simulink model "gm_whdlOFDMTx"  (R2022b)
settings: Solver=FixedStepDiscrete  StartTime=0.0  StopTime=0  RelTol=1e-3
model workspace (MATLAB code in the model file):
  | config = whdlexamples.OFDMTxParameters();
  | fftLen = config.fftLen;
  | subC = config.subC;
  | cpLen = config.cpLen;
  | fs = config.fs;
  | NSS = config.NSS;
  | NRS = config.NRS;
  | NHeader = config.NHeader;
  | NData = config.NData;
  | NSymPerF = config.NSymPerF;
  | ssSymbol = config.ssSymbol;
  | rsSymbol = config.rsSymbol;
  | NHeaderBits = config.NHeaderBits;
  | headerCRCBool = config.headerCRCBool;
  | headerConvK = config.headerConvK;
  | headerConvCode = config.headerConvCode;
  | pilotValPerSym = config.pilotValPerSym;
  | pilotLen = config.pilotLen;
  | dataCRCPoly = config.dataCRCPoly;
  | dataCRCBool = config.dataCRCBool;
  | dataCRCLen = config.dataCRCLen;
  | dataConvK = config.dataConvK;
  | dataConvCode = config.dataConvCode;
  | scramInit = config.scramInit;
  | firCoeff = config.firCoeff;
  | rateFac1 = config.rateFac1;
  | rateFac2 = config.rateFac2;
  | headerLat = config.headerLat;
  | headerTime = config.headerTime;
  | preambleInd = config.preambleInd;
  | headerDataInd = config.headerDataInd;
  | trBlkSize = config.trBlkSize;
  | randOFDM = config.randOFDM;
  | headerIntrlvMaxBlkSize = config.headerIntrlvMaxBlkSize;
  | headerIntrlvNColumns   = config.headerIntrlvNColumns;
  | dataIntrlvMaxBlkSize   = config.dataIntrlvMaxBlkSize;
  | dataIntrlvNColumns     = config.dataIntrlvNColumns;
  | clear config
libraries: hdlsllib x49, simulink x22, dspsigops x11, whdlmod x3, whdledac x3, whdlutilities x2, commhdlcrc x2, dsphdlfiltering2 x1
(part 3 of 4)

== system gm_whdlOFDMTx/Frame Generator/Header/Interleaver/Read Logic/Generate Base Read Address ==
  readStart : Inport  OutDataTypeStr=boolean  PortDimensions=1  SampleTime=2.44140625e-07
  Constant1 : Constant  Value=0  OutDataTypeStr=fixdt(0,nextpow2(maxBlkSize+1),0)  SampleTime=-1
  Constant5 : Constant  Value=maxBlkSize  OutDataTypeStr=fixdt(0,nextpow2(maxBlkSize+1),0)  SampleTime=-1
  Logical Operator7 : Logic  Operator=NOT  IconShape=distinctive  AllPortsSameDT=off  OutDataTypeStr=boolean
  Switch1 : Switch  Criteria=u2 ~= 0  SaturateOnIntegerOverflow=off  InputSameDT=off
  Unit Delay Enabled Synchronous2 : hdlsllib/Discrete/Unit Delay Enabled Synchronous  InitialCondition=1  SampleTime=-1
  baseAddr : Outport  SampleTime=2.44140625e-07
  wires:
  readStart/1 -> Unit Delay Enabled Synchronous2/2
  Constant1/1 -> Switch1/3
  Constant5/1 -> Switch1/1
  Logical Operator7/1 -> Unit Delay Enabled Synchronous2/1
  Switch1/1 -> baseAddr/1
  Unit Delay Enabled Synchronous2/1 -> Switch1/2, Logical Operator7/1

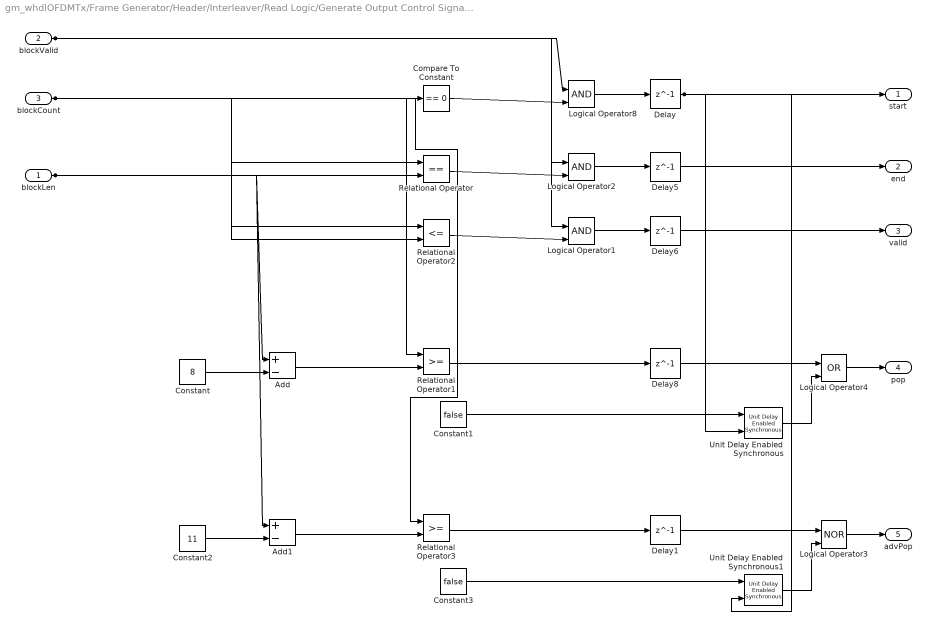
== system gm_whdlOFDMTx/Frame Generator/Header/Interleaver/Read Logic/Generate Output Control Signals ==
  blockLen : Inport  OutDataTypeStr=fixdt(0, 7, 0)  PortDimensions=1  SampleTime=2.44140625e-07
  blockValid : Inport  Port=2  OutDataTypeStr=boolean  PortDimensions=1  SampleTime=2.44140625e-07
  blockCount : Inport  Port=3  OutDataTypeStr=fixdt(0, 7, 0)  PortDimensions=1  SampleTime=2.44140625e-07
  Add : Sum  Inputs=+-
  Add1 : Sum  Inputs=+-
  Compare To Constant : simulink/Logic and Bit Operations/Compare To Constant  relop===  const=0  OutDataTypeStr=boolean
  Constant : Constant  Value=8  OutDataTypeStr=fixdt(0,nextpow2(8+1),0)  SampleTime=-1
  Constant1 : Constant  Value=false  SampleTime=-1
  Constant2 : Constant  Value=11  OutDataTypeStr=fixdt(0,nextpow2(11+1),0)  SampleTime=-1
  Constant3 : Constant  Value=false  SampleTime=-1
  Delay{,1,5..6,8} (5 alike) : Delay  DelayLength=1
  Logical Operator1 : Logic  IconShape=distinctive  AllPortsSameDT=off  OutDataTypeStr=boolean
  Logical Operator2 : Logic  IconShape=distinctive  AllPortsSameDT=off  OutDataTypeStr=boolean
  Logical Operator3 : Logic  Operator=NOR  IconShape=distinctive  AllPortsSameDT=off  OutDataTypeStr=boolean
  Logical Operator4 : Logic  Operator=OR  IconShape=distinctive  AllPortsSameDT=off  OutDataTypeStr=boolean
  Logical Operator8 : Logic  IconShape=distinctive  AllPortsSameDT=off  OutDataTypeStr=boolean
  Relational Operator : RelationalOperator  Operator===  OutDataTypeStr=boolean  InputSameDT=off
  Relational Operator1 : RelationalOperator  OutDataTypeStr=boolean  InputSameDT=off
  Relational Operator2 : RelationalOperator  Operator=<=  OutDataTypeStr=boolean  InputSameDT=off
  Relational Operator3 : RelationalOperator  OutDataTypeStr=boolean  InputSameDT=off
  Unit Delay Enabled Synchronous : hdlsllib/Discrete/Unit Delay Enabled Synchronous  InitialCondition=1  SampleTime=-1
  Unit Delay Enabled Synchronous1 : hdlsllib/Discrete/Unit Delay Enabled Synchronous  InitialCondition=1  SampleTime=-1
  start : Outport  SampleTime=2.44140625e-07
  end : Outport  Port=2  SampleTime=2.44140625e-07
  valid : Outport  Port=3  SampleTime=2.44140625e-07
  pop : Outport  Port=4  SampleTime=2.44140625e-07
  advPop : Outport  Port=5  SampleTime=2.44140625e-07
  wires:
  blockLen/1 -> Relational Operator2/2, Relational Operator/2, Add1/1, Add/1
  blockValid/1 -> Logical Operator8/1, Logical Operator2/1, Logical Operator1/1
  blockCount/1 -> Relational Operator3/1, Relational Operator2/1, Relational Operator1/1, Relational Operator/1, Compare To Constant/1
  Add/1 -> Relational Operator1/2
  Add1/1 -> Relational Operator3/2
  Compare To Constant/1 -> Logical Operator8/2
  Constant/1 -> Add/2
  Constant1/1 -> Unit Delay Enabled Synchronous/1
  Constant2/1 -> Add1/2
  Constant3/1 -> Unit Delay Enabled Synchronous1/1
  Delay/1 -> Unit Delay Enabled Synchronous1/2, Unit Delay Enabled Synchronous/2, start/1
  Delay1/1 -> Logical Operator3/1
  Delay5/1 -> end/1
  Delay6/1 -> valid/1
  Delay8/1 -> Logical Operator4/1
  Logical Operator1/1 -> Delay6/1
  Logical Operator2/1 -> Delay5/1
  Logical Operator3/1 -> advPop/1
  Logical Operator4/1 -> pop/1
  Logical Operator8/1 -> Delay/1
  Relational Operator/1 -> Logical Operator2/2
  Relational Operator1/1 -> Delay8/1
  Relational Operator2/1 -> Logical Operator1/2
  Relational Operator3/1 -> Delay1/1
  Unit Delay Enabled Synchronous/1 -> Logical Operator4/2
  Unit Delay Enabled Synchronous1/1 -> Logical Operator3/2

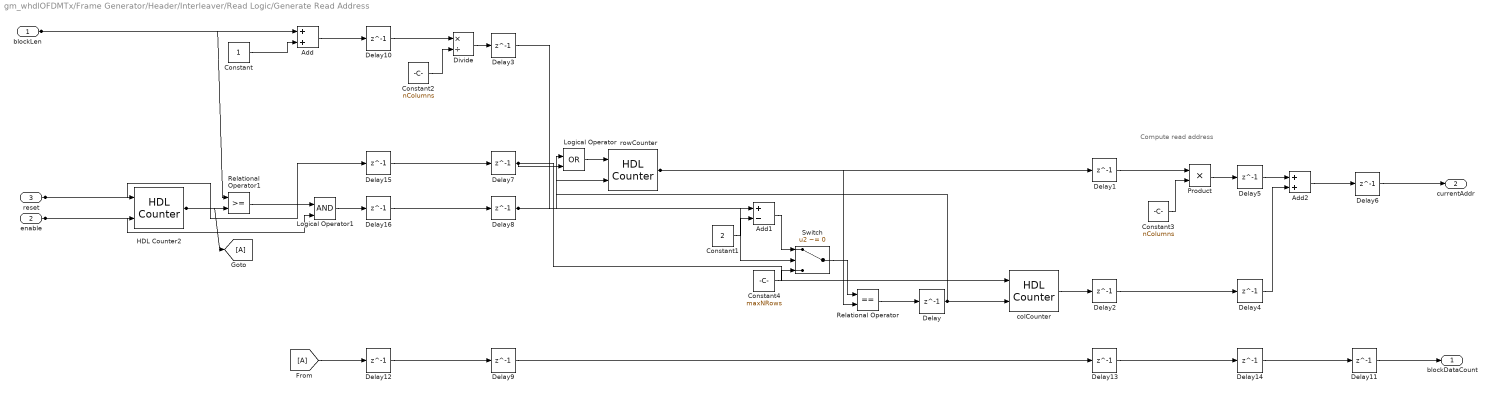
== system gm_whdlOFDMTx/Frame Generator/Header/Interleaver/Read Logic/Generate Read Address ==
  note: Compute read address
  blockLen : Inport  OutDataTypeStr=fixdt(0, 7, 0)  PortDimensions=1  SampleTime=2.44140625e-07
  enable : Inport  Port=2  OutDataTypeStr=boolean  PortDimensions=1  SampleTime=2.44140625e-07
  reset : Inport  Port=3  OutDataTypeStr=boolean  PortDimensions=1  SampleTime=2.44140625e-07
  Add : Sum
  Add1 : Sum  Inputs=+-  OutDataTypeStr=Inherit: Inherit via back propagation
  Add2 : Sum  OutDataTypeStr=fixdt(0,nextpow2(maxBlkSize),0)
  Constant : Constant  OutDataTypeStr=fixdt(0,1,0)  SampleTime=-1
  Constant1 : Constant  Value=2  OutDataTypeStr=fixdt(0,2,0)  SampleTime=-1
  Constant2 : Constant  Value=nColumns  OutDataTypeStr=fixdt(0,nextpow2(nColumns+1),0)  SampleTime=-1
  Constant3 : Constant  Value=nColumns  OutDataTypeStr=fixdt(0,nextpow2(nColumns+1),0)  SampleTime=-1
  Constant4 : Constant  Value=maxNRows  OutDataTypeStr=Inherit: Inherit via back propagation  SampleTime=-1
  Delay{,1..16} (17 alike) : Delay  DelayLength=1
  Divide : Product  Inputs=*/  OutDataTypeStr=fixdt(0,nextpow2(maxNRows+1),0)  RndMeth=Zero  SaturateOnIntegerOverflow=on
  From : From
  Goto : Goto
  HDL Counter2 : hdlsllib/Sources/HDL Counter  CountType=Count limited  CountInit=0  CountStep=1  CountMax=maxBlkSize  CountFromType=Initial value  CountFrom=0  CountResetPort=on  CountLoadPort=off  CountEnbPort=on  CountDirPort=off  CountHitOutputPort=off  CountDataType=Unsigned  CountWordLen=nextpow2(maxBlkSize+1)  CountFracLen=0  CountSampTime=1
  Logical Operator : Logic  Operator=OR  IconShape=distinctive  AllPortsSameDT=off  OutDataTypeStr=boolean
  Logical Operator1 : Logic  IconShape=distinctive  AllPortsSameDT=off  OutDataTypeStr=boolean
  Product : Product  OutDataTypeStr=fixdt(0,nextpow2(maxBlkSize),0)
  Relational Operator : RelationalOperator  Operator===  OutDataTypeStr=boolean  InputSameDT=off
  Relational Operator1 : RelationalOperator  OutDataTypeStr=boolean  InputSameDT=off
  Switch : Switch  Criteria=u2 ~= 0  SaturateOnIntegerOverflow=off  InputSameDT=off
  colCounter : hdlsllib/Sources/HDL Counter  CountType=Count limited  CountInit=0  CountStep=1  CountMax=nColumns -1  CountFromType=Initial value  CountFrom=0  CountResetPort=on  CountLoadPort=off  CountEnbPort=on  CountDirPort=off  CountHitOutputPort=off  CountDataType=Unsigned  CountWordLen=nextpow2(nColumns)  CountFracLen=0  CountSampTime=1
  rowCounter : hdlsllib/Sources/HDL Counter  CountType=Count limited  CountInit=0  CountStep=1  CountMax=maxNRows -1  CountFromType=Initial value  CountFrom=0  CountResetPort=on  CountLoadPort=off  CountEnbPort=on  CountDirPort=off  CountHitOutputPort=off  CountDataType=Unsigned  CountWordLen=nextpow2(maxNRows+1)  CountFracLen=0  CountSampTime=1
  blockDataCount : Outport  SampleTime=2.44140625e-07
  currentAddr : Outport  Port=2  SampleTime=2.44140625e-07
  wires:
  blockLen/1 -> Relational Operator1/1, Add/1
  enable/1 -> Logical Operator1/2, HDL Counter2/2
  reset/1 -> Delay15/1, HDL Counter2/1
  Add/1 -> Delay10/1
  Add1/1 -> Switch/1
  Add2/1 -> Delay6/1
  Constant/1 -> Add/2
  Constant1/1 -> Add1/2
  Constant2/1 -> Divide/2
  Constant3/1 -> Product/2
  Constant4/1 -> Switch/3
  Delay/1 -> Logical Operator/1, colCounter/2
  Delay1/1 -> Product/1
  Delay10/1 -> Divide/1
  Delay11/1 -> blockDataCount/1
  Delay12/1 -> Delay9/1
  Delay13/1 -> Delay14/1
  Delay14/1 -> Delay11/1
  Delay15/1 -> Delay7/1
  Delay16/1 -> Delay8/1
  Delay2/1 -> Delay4/1
  Delay3/1 -> Add1/1
  Delay4/1 -> Add2/2
  Delay5/1 -> Add2/1
  Delay6/1 -> currentAddr/1
  Delay7/1 -> Logical Operator/2, colCounter/1
  Delay8/1 -> Switch/2, rowCounter/2
  Delay9/1 -> Delay13/1
  Divide/1 -> Delay3/1
  From/1 -> Delay12/1
  HDL Counter2/1 -> Relational Operator1/2, Goto/1
  Logical Operator/1 -> rowCounter/1
  Logical Operator1/1 -> Delay16/1
  Product/1 -> Delay5/1
  Relational Operator/1 -> Delay/1
  Relational Operator1/1 -> Logical Operator1/1
  Switch/1 -> Relational Operator/1
  colCounter/1 -> Delay2/1
  rowCounter/1 -> Relational Operator/2, Delay1/1

== system gm_whdlOFDMTx/Frame Generator/Header/Interleaver/Read Logic/MATLAB Function ==
  trigger : Inport  OutDataTypeStr=boolean  PortDimensions=1  SampleTime=2.44140625e-07
  MATLAB Function : MATLAB Function  TreatAsAtomicUnit=on  mask{nClocks=maxBlkSize}
      mask prompts: nClocks "Number of clocks to hold:"
  out : Outport  SampleTime=2.44140625e-07  VectorParamsAs1DForOutWhenUnconnected=off
  wires:
  trigger/1 -> MATLAB Function/1(trigger)
  MATLAB Function/1(out) -> out/1

== system gm_whdlOFDMTx/Frame Generator/Header/Interleaver/Write Logic/Generate Write Address ==
  rst : Inport  OutDataTypeStr=boolean  PortDimensions=1  SampleTime=2.44140625e-07
  enb : Inport  Port=2  OutDataTypeStr=boolean  PortDimensions=1  SampleTime=2.44140625e-07
  end : Inport  Port=3  OutDataTypeStr=boolean  PortDimensions=1  SampleTime=2.44140625e-07
  Add : Sum  OutDataTypeStr=Inherit: Inherit via back propagation
  Constant : Constant  Value=0  OutDataTypeStr=fixdt(0,nextpow2(maxBlkSize+1),0)  SampleTime=-1
  Constant4 : Constant  Value=maxBlkSize  OutDataTypeStr=fixdt(0,nextpow2(maxBlkSize+1),0)  SampleTime=-1
  HDL Counter : hdlsllib/Sources/HDL Counter  CountType=Count limited  CountInit=0  CountStep=1  CountMax=maxBlkSize  CountFromType=Initial value  CountFrom=0  CountResetPort=on  CountLoadPort=off  CountEnbPort=on  CountDirPort=off  CountHitOutputPort=off  CountDataType=Unsigned  CountWordLen=nextpow2(maxBlkSize+1)  CountFracLen=0  CountSampTime=1
  Logical Operator7 : Logic  Operator=NOT  IconShape=distinctive  AllPortsSameDT=off  OutDataTypeStr=boolean
  Switch : Switch  Criteria=u2 ~= 0  SaturateOnIntegerOverflow=off  InputSameDT=off
  Unit Delay Enabled Synchronous2 : hdlsllib/Discrete/Unit Delay Enabled Synchronous  InitialCondition=0  SampleTime=-1
  wrAddr : Outport  SampleTime=2.44140625e-07
  count : Outport  Port=2  SampleTime=2.44140625e-07
  wires:
  rst/1 -> HDL Counter/1
  enb/1 -> HDL Counter/2
  end/1 -> Unit Delay Enabled Synchronous2/2
  Add/1 -> wrAddr/1
  Constant/1 -> Switch/3
  Constant4/1 -> Switch/1
  HDL Counter/1 -> Add/1, count/1
  Logical Operator7/1 -> Unit Delay Enabled Synchronous2/1
  Switch/1 -> Add/2
  Unit Delay Enabled Synchronous2/1 -> Switch/2, Logical Operator7/1

== system gm_whdlOFDMTx/Frame Generator/Header/Interleaver/Write Logic/Handle Input Control Signals ==
  start : Inport  OutDataTypeStr=boolean  PortDimensions=1  SampleTime=2.44140625e-07
  valid : Inport  Port=2  OutDataTypeStr=boolean  PortDimensions=1  SampleTime=2.44140625e-07
  end : Inport  Port=3  OutDataTypeStr=boolean  PortDimensions=1  SampleTime=2.44140625e-07
  Delay{1..5} (5 alike) : Delay  DelayLength=1
  Generate Current Frame Status : Subsystem
  Generate Forced End : Subsystem
  Logical Operator : Logic  Operator=OR  IconShape=distinctive  AllPortsSameDT=off  OutDataTypeStr=boolean
  Logical Operator1 : Logic  Operator=NOT  IconShape=distinctive  AllPortsSameDT=off  OutDataTypeStr=boolean
  Logical Operator2 : Logic  IconShape=distinctive  AllPortsSameDT=off  OutDataTypeStr=boolean
  Logical Operator3 : Logic  Inputs=4  IconShape=distinctive  AllPortsSameDT=off  OutDataTypeStr=boolean
  Logical Operator5 : Logic  IconShape=distinctive  AllPortsSameDT=off  OutDataTypeStr=boolean
  reset : Outport  SampleTime=2.44140625e-07
  countEnb : Outport  Port=2  SampleTime=2.44140625e-07
  endOut : Outport  Port=3  SampleTime=2.44140625e-07
  endReady : Outport  Port=4  SampleTime=2.44140625e-07
  wires:
  start/1 -> Logical Operator2/1
  valid/1 -> Logical Operator3/1, Logical Operator2/2, Delay4/1, Generate Forced End/2(valid)
  end/1 -> Logical Operator3/2
  Delay1/1 -> Logical Operator1/1, Delay5/1, Generate Current Frame Status/2(end)
  Delay2/1 -> reset/1
  Delay3/1 -> countEnb/1
  Delay4/1 -> Logical Operator5/1
  Delay5/1 -> endOut/1
  Generate Current Frame Status/1(frameOn) -> Logical Operator5/2, Logical Operator3/3, Generate Forced End/3(frameOn)
  Generate Forced End/1(forcedEnd) -> Logical Operator/2
  Logical Operator/1 -> Delay1/1, endReady/1
  Logical Operator1/1 -> Logical Operator3/4
  Logical Operator2/1 -> Delay2/1, Generate Current Frame Status/1(start), Generate Forced End/1(rst)
  Logical Operator3/1 -> Logical Operator/1
  Logical Operator5/1 -> Delay3/1

== system gm_whdlOFDMTx/Frame Controller and Input Sampler/Frame Controller/Generate OFDM Modulator Ready/Control OFDM Signal Generation/Disable OFDM Generation/MATLAB Function5 ==
  trigger : Inport  OutDataTypeStr=boolean  PortDimensions=1  SampleTime=4.8828125e-07
  MATLAB Function5 : MATLAB Function  TreatAsAtomicUnit=on  mask{nClocks=(fftLen+cpLen)*rateFac2 -1}
      mask prompts: nClocks "Number of clocks to hold:"
  out : Outport  SampleTime=4.8828125e-07  VectorParamsAs1DForOutWhenUnconnected=off
  wires:
  trigger/1 -> MATLAB Function5/1(trigger)
  MATLAB Function5/1(out) -> out/1

== system gm_whdlOFDMTx/Frame Generator/Data/Data Chain/Symbol Interleaver/Interleaver/Generate Ready ==
  advPop : Inport  OutDataTypeStr=boolean  PortDimensions=1  SampleTime=2.44140625e-07
  fifoCount : Inport  Port=2  OutDataTypeStr=fixdt(0, 3, 0)  PortDimensions=1  SampleTime=2.44140625e-07
  pop : Inport  Port=3  OutDataTypeStr=boolean  PortDimensions=1  SampleTime=2.44140625e-07
  endReady : Inport  Port=4  OutDataTypeStr=boolean  PortDimensions=1  SampleTime=2.44140625e-07
  Generate Ready2 : Subsystem
  Logical Operator1 : Logic  IconShape=distinctive  AllPortsSameDT=off  OutDataTypeStr=boolean
  Logical Operator2 : Logic  IconShape=distinctive  AllPortsSameDT=off  OutDataTypeStr=boolean
  Logical Operator3 : Logic  Operator=NOT  IconShape=distinctive  AllPortsSameDT=off  OutDataTypeStr=boolean
  MATLAB Function1 : Subsystem
  ready : Outport  SampleTime=2.44140625e-07
  wires:
  advPop/1 -> Logical Operator1/1
  fifoCount/1 -> Generate Ready2/1(fifoCount)
  pop/1 -> Generate Ready2/2(pop)
  endReady/1 -> Logical Operator1/2
  Generate Ready2/1(ready2) -> Logical Operator2/1
  Logical Operator1/1 -> MATLAB Function1/1(trigger)
  Logical Operator2/1 -> ready/1
  Logical Operator3/1 -> Logical Operator2/2
  MATLAB Function1/1(out) -> Logical Operator3/1

== system gm_whdlOFDMTx/Frame Generator/Data/Data Chain/Symbol Interleaver/Interleaver/Read Logic ==
  fifoData : Inport  OutDataTypeStr=fixdt(0, 9, 0)  PortDimensions=1  SampleTime=2.44140625e-07
  fifoCount : Inport  Port=2  OutDataTypeStr=fixdt(0, 3, 0)  PortDimensions=1  SampleTime=2.44140625e-07
  Add1 : Sum  OutDataTypeStr=Inherit: Inherit via back propagation
  Delay1 : Delay  DelayLength=5
  Delay2 : Delay  DelayLength=5
  Delay3 : Delay  DelayLength=1
  Delay4 : Delay  DelayLength=5
  Delay7 : Delay  DelayLength=1
  Generate Base Read Address : Subsystem
  Generate Output Control Signals : Subsystem
  Generate Read Address : Subsystem
  MATLAB Function : Subsystem
  Relational Operator1 : RelationalOperator  Operator=<  OutDataTypeStr=boolean  InputSameDT=off
  Unit Delay Enabled Synchronous1 : hdlsllib/Discrete/Unit Delay Enabled Synchronous  InitialCondition=maxBlkSize -1  SampleTime=-1
  rdAddr : Outport  SampleTime=2.44140625e-07
  start : Outport  Port=2  SampleTime=2.44140625e-07
  end : Outport  Port=3  SampleTime=2.44140625e-07
  valid : Outport  Port=4  SampleTime=2.44140625e-07
  pop : Outport  Port=5  SampleTime=2.44140625e-07
  advPop : Outport  Port=6  SampleTime=2.44140625e-07
  wires:
  fifoData/1 -> Unit Delay Enabled Synchronous1/1
  fifoCount/1 -> Relational Operator1/1, Delay3/1
  Add1/1 -> Delay7/1
  Delay1/1 -> Add1/2
  Delay2/1 -> Generate Output Control Signals/2(blockValid)
  Delay3/1 -> Relational Operator1/2
  Delay4/1 -> Generate Output Control Signals/1(blockLen)
  Delay7/1 -> rdAddr/1
  Generate Base Read Address/1(baseAddr) -> Delay1/1
  Generate Output Control Signals/1(start) -> start/1
  Generate Output Control Signals/2(end) -> end/1
  Generate Output Control Signals/3(valid) -> valid/1
  Generate Output Control Signals/4(pop) -> pop/1
  Generate Output Control Signals/5(advPop) -> advPop/1
  Generate Read Address/1(blockDataCount) -> Generate Output Control Signals/3(blockCount)
  Generate Read Address/2(currentAddr) -> Add1/1
  MATLAB Function/1(out) -> Delay2/1, Generate Read Address/2(enable)
  Relational Operator1/1 -> Unit Delay Enabled Synchronous1/2, MATLAB Function/1(trigger), Generate Read Address/3(reset), Generate Base Read Address/1(readStart)
  Unit Delay Enabled Synchronous1/1 -> Delay4/1, Generate Read Address/1(blockLen)

== system gm_whdlOFDMTx/Frame Generator/Data/Data Chain/Symbol Interleaver/Interleaver/Write Logic ==
  start : Inport  OutDataTypeStr=boolean  PortDimensions=1  SampleTime=2.44140625e-07
  valid : Inport  Port=2  OutDataTypeStr=boolean  PortDimensions=1  SampleTime=2.44140625e-07
  end : Inport  Port=3  OutDataTypeStr=boolean  PortDimensions=1  SampleTime=2.44140625e-07
  Generate Write Address : Subsystem
  Handle Input Control Signals : Subsystem
  wrAddr : Outport  SampleTime=2.44140625e-07
  wrValid : Outport  Port=2  SampleTime=2.44140625e-07
  count : Outport  Port=3  SampleTime=2.44140625e-07
  endOut : Outport  Port=4  SampleTime=2.44140625e-07
  endReady : Outport  Port=5  SampleTime=2.44140625e-07
  wires:
  start/1 -> Handle Input Control Signals/1(start)
  valid/1 -> Handle Input Control Signals/2(valid)
  end/1 -> Handle Input Control Signals/3(end)
  Generate Write Address/1(wrAddr) -> wrAddr/1
  Generate Write Address/2(count) -> count/1
  Handle Input Control Signals/1(reset) -> Generate Write Address/1(rst)
  Handle Input Control Signals/2(countEnb) -> wrValid/1, Generate Write Address/2(enb)
  Handle Input Control Signals/3(endOut) -> endOut/1, Generate Write Address/3(end)
  Handle Input Control Signals/4(endReady) -> endReady/1

== system gm_whdlOFDMTx/Frame Generator/Header/Interleaver/Write Logic/Handle Input Control Signals/Generate Current Frame Status ==
  start : Inport  OutDataTypeStr=boolean  PortDimensions=1  SampleTime=2.44140625e-07
  end : Inport  Port=2  OutDataTypeStr=boolean  PortDimensions=1  SampleTime=2.44140625e-07
  Constant2 : Constant  Value=true  OutDataTypeStr=Inherit: Inherit via back propagation  SampleTime=-1
  Constant3 : Constant  Value=false  OutDataTypeStr=Inherit: Inherit via back propagation  SampleTime=-1
  Delay3 : Delay  DelayLength=1
  Logical Operator4 : Logic  Operator=OR  IconShape=distinctive  AllPortsSameDT=off  OutDataTypeStr=boolean
  Logical Operator6 : Logic  IconShape=distinctive  AllPortsSameDT=off  OutDataTypeStr=boolean
  Logical Operator7 : Logic  Operator=NOT  IconShape=distinctive  AllPortsSameDT=off  OutDataTypeStr=boolean
  Switch2 : Switch  Criteria=u2 ~= 0  SaturateOnIntegerOverflow=off  InputSameDT=off
  Unit Delay Enabled Synchronous1 : hdlsllib/Discrete/Unit Delay Enabled Synchronous  InitialCondition=0  SampleTime=-1
  frameOn : Outport  SampleTime=2.44140625e-07
  wires:
  start/1 -> Switch2/2, Logical Operator4/1, Delay3/1
  end/1 -> Logical Operator6/2
  Constant2/1 -> Switch2/1
  Constant3/1 -> Switch2/3
  Delay3/1 -> Logical Operator7/1
  Logical Operator4/1 -> Unit Delay Enabled Synchronous1/2
  Logical Operator6/1 -> Logical Operator4/2
  Logical Operator7/1 -> Logical Operator6/1
  Switch2/1 -> Unit Delay Enabled Synchronous1/1
  Unit Delay Enabled Synchronous1/1 -> frameOn/1

== system gm_whdlOFDMTx/Frame Generator/Header/Interleaver/Write Logic/Handle Input Control Signals/Generate Forced End ==
  rst : Inport  OutDataTypeStr=boolean  PortDimensions=1  SampleTime=2.44140625e-07
  valid : Inport  Port=2  OutDataTypeStr=boolean  PortDimensions=1  SampleTime=2.44140625e-07
  frameOn : Inport  Port=3  OutDataTypeStr=boolean  PortDimensions=1  SampleTime=2.44140625e-07
  Compare To Constant1 : simulink/Logic and Bit Operations/Compare To Constant  relop===  const=maxBlkSize -2  OutDataTypeStr=boolean
  Logical Operator1 : Logic  IconShape=distinctive  AllPortsSameDT=off  OutDataTypeStr=boolean
  Logical Operator6 : Logic  IconShape=distinctive  AllPortsSameDT=off  OutDataTypeStr=boolean
  readyCounter : hdlsllib/Sources/HDL Counter  CountType=Count limited  CountInit=0  CountStep=1  CountMax=maxBlkSize  CountFromType=Initial value  CountFrom=0  CountResetPort=on  CountLoadPort=off  CountEnbPort=on  CountDirPort=off  CountHitOutputPort=off  CountDataType=Unsigned  CountWordLen=nextpow2(maxBlkSize+1)  CountFracLen=0  CountSampTime=1
  forcedEnd : Outport  SampleTime=2.44140625e-07
  wires:
  rst/1 -> readyCounter/1
  valid/1 -> Logical Operator1/1
  frameOn/1 -> Logical Operator1/2
  Compare To Constant1/1 -> Logical Operator6/1
  Logical Operator1/1 -> Logical Operator6/2, readyCounter/2
  Logical Operator6/1 -> forcedEnd/1
  readyCounter/1 -> Compare To Constant1/1

== system gm_whdlOFDMTx/Frame Generator/Data/Data Chain/Symbol Interleaver/Interleaver/Generate Ready/Generate Ready2 ==
  fifoCount : Inport  OutDataTypeStr=fixdt(0, 3, 0)  PortDimensions=1  SampleTime=2.44140625e-07
  pop : Inport  Port=2  OutDataTypeStr=boolean  PortDimensions=1  SampleTime=2.44140625e-07
  Compare To Constant1 : simulink/Logic and Bit Operations/Compare To Constant  relop===  const=0  OutDataTypeStr=boolean
  Compare To Constant4 : simulink/Logic and Bit Operations/Compare To Constant  relop===  const=1  OutDataTypeStr=boolean
  Logical Operator1 : Logic  Operator=OR  IconShape=distinctive  AllPortsSameDT=off  OutDataTypeStr=boolean
  Logical Operator14 : Logic  IconShape=distinctive  AllPortsSameDT=off  OutDataTypeStr=boolean
  ready2 : Outport  SampleTime=2.44140625e-07
  wires:
  fifoCount/1 -> Compare To Constant4/1, Compare To Constant1/1
  pop/1 -> Logical Operator14/2
  Compare To Constant1/1 -> Logical Operator1/1
  Compare To Constant4/1 -> Logical Operator14/1
  Logical Operator1/1 -> ready2/1
  Logical Operator14/1 -> Logical Operator1/2

== system gm_whdlOFDMTx/Frame Generator/Data/Data Chain/Symbol Interleaver/Interleaver/Generate Ready/MATLAB Function1 ==
  trigger : Inport  OutDataTypeStr=boolean  PortDimensions=1  SampleTime=2.44140625e-07
  MATLAB Function1 : MATLAB Function  TreatAsAtomicUnit=on  mask{nClocks=4}
      mask prompts: nClocks "Number of clocks to hold:"
  out : Outport  SampleTime=2.44140625e-07  VectorParamsAs1DForOutWhenUnconnected=off
  wires:
  trigger/1 -> MATLAB Function1/1(trigger)
  MATLAB Function1/1(out) -> out/1

== system gm_whdlOFDMTx/Frame Generator/Data/Data Chain/Symbol Interleaver/Interleaver/Read Logic/Generate Base Read Address ==
  readStart : Inport  OutDataTypeStr=boolean  PortDimensions=1  SampleTime=2.44140625e-07
  Constant1 : Constant  Value=0  OutDataTypeStr=fixdt(0,nextpow2(maxBlkSize+1),0)  SampleTime=-1
  Constant5 : Constant  Value=maxBlkSize  OutDataTypeStr=fixdt(0,nextpow2(maxBlkSize+1),0)  SampleTime=-1
  Logical Operator7 : Logic  Operator=NOT  IconShape=distinctive  AllPortsSameDT=off  OutDataTypeStr=boolean
  Switch1 : Switch  Criteria=u2 ~= 0  SaturateOnIntegerOverflow=off  InputSameDT=off
  Unit Delay Enabled Synchronous2 : hdlsllib/Discrete/Unit Delay Enabled Synchronous  InitialCondition=1  SampleTime=-1
  baseAddr : Outport  SampleTime=2.44140625e-07
  wires:
  readStart/1 -> Unit Delay Enabled Synchronous2/2
  Constant1/1 -> Switch1/3
  Constant5/1 -> Switch1/1
  Logical Operator7/1 -> Unit Delay Enabled Synchronous2/1
  Switch1/1 -> baseAddr/1
  Unit Delay Enabled Synchronous2/1 -> Switch1/2, Logical Operator7/1

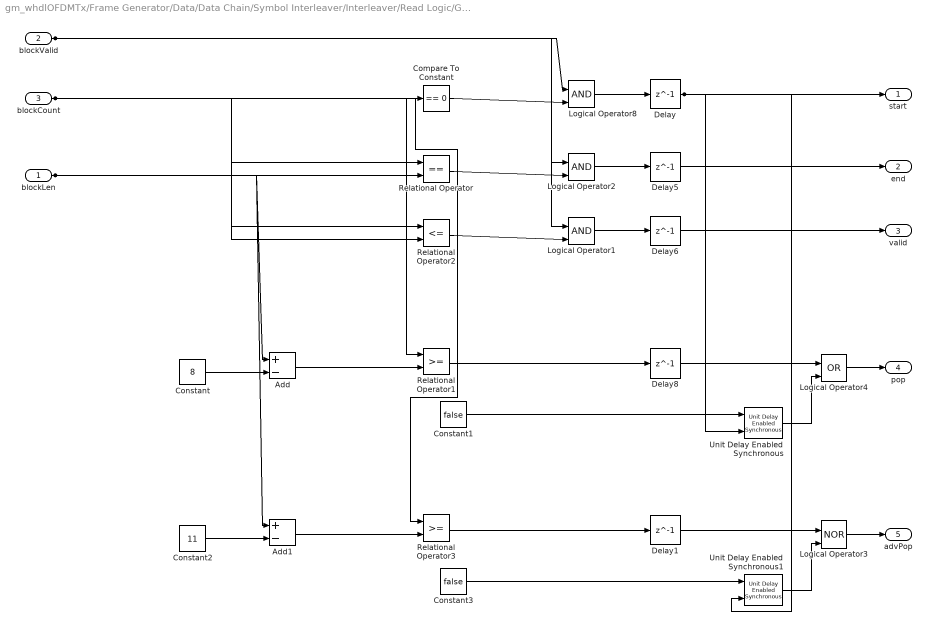
== system gm_whdlOFDMTx/Frame Generator/Data/Data Chain/Symbol Interleaver/Interleaver/Read Logic/Generate Output Control Signals ==
  blockLen : Inport  OutDataTypeStr=fixdt(0, 9, 0)  PortDimensions=1  SampleTime=2.44140625e-07
  blockValid : Inport  Port=2  OutDataTypeStr=boolean  PortDimensions=1  SampleTime=2.44140625e-07
  blockCount : Inport  Port=3  OutDataTypeStr=fixdt(0, 9, 0)  PortDimensions=1  SampleTime=2.44140625e-07
  Add : Sum  Inputs=+-
  Add1 : Sum  Inputs=+-
  Compare To Constant : simulink/Logic and Bit Operations/Compare To Constant  relop===  const=0  OutDataTypeStr=boolean
  Constant : Constant  Value=8  OutDataTypeStr=fixdt(0,nextpow2(8+1),0)  SampleTime=-1
  Constant1 : Constant  Value=false  SampleTime=-1
  Constant2 : Constant  Value=11  OutDataTypeStr=fixdt(0,nextpow2(11+1),0)  SampleTime=-1
  Constant3 : Constant  Value=false  SampleTime=-1
  Delay{,1,5..6,8} (5 alike) : Delay  DelayLength=1
  Logical Operator1 : Logic  IconShape=distinctive  AllPortsSameDT=off  OutDataTypeStr=boolean
  Logical Operator2 : Logic  IconShape=distinctive  AllPortsSameDT=off  OutDataTypeStr=boolean
  Logical Operator3 : Logic  Operator=NOR  IconShape=distinctive  AllPortsSameDT=off  OutDataTypeStr=boolean
  Logical Operator4 : Logic  Operator=OR  IconShape=distinctive  AllPortsSameDT=off  OutDataTypeStr=boolean
  Logical Operator8 : Logic  IconShape=distinctive  AllPortsSameDT=off  OutDataTypeStr=boolean
  Relational Operator : RelationalOperator  Operator===  OutDataTypeStr=boolean  InputSameDT=off
  Relational Operator1 : RelationalOperator  OutDataTypeStr=boolean  InputSameDT=off
  Relational Operator2 : RelationalOperator  Operator=<=  OutDataTypeStr=boolean  InputSameDT=off
  Relational Operator3 : RelationalOperator  OutDataTypeStr=boolean  InputSameDT=off
  Unit Delay Enabled Synchronous : hdlsllib/Discrete/Unit Delay Enabled Synchronous  InitialCondition=1  SampleTime=-1
  Unit Delay Enabled Synchronous1 : hdlsllib/Discrete/Unit Delay Enabled Synchronous  InitialCondition=1  SampleTime=-1
  start : Outport  SampleTime=2.44140625e-07
  end : Outport  Port=2  SampleTime=2.44140625e-07
  valid : Outport  Port=3  SampleTime=2.44140625e-07
  pop : Outport  Port=4  SampleTime=2.44140625e-07
  advPop : Outport  Port=5  SampleTime=2.44140625e-07
  wires:
  blockLen/1 -> Relational Operator2/2, Relational Operator/2, Add1/1, Add/1
  blockValid/1 -> Logical Operator8/1, Logical Operator2/1, Logical Operator1/1
  blockCount/1 -> Relational Operator3/1, Relational Operator2/1, Relational Operator1/1, Relational Operator/1, Compare To Constant/1
  Add/1 -> Relational Operator1/2
  Add1/1 -> Relational Operator3/2
  Compare To Constant/1 -> Logical Operator8/2
  Constant/1 -> Add/2
  Constant1/1 -> Unit Delay Enabled Synchronous/1
  Constant2/1 -> Add1/2
  Constant3/1 -> Unit Delay Enabled Synchronous1/1
  Delay/1 -> Unit Delay Enabled Synchronous1/2, Unit Delay Enabled Synchronous/2, start/1
  Delay1/1 -> Logical Operator3/1
  Delay5/1 -> end/1
  Delay6/1 -> valid/1
  Delay8/1 -> Logical Operator4/1
  Logical Operator1/1 -> Delay6/1
  Logical Operator2/1 -> Delay5/1
  Logical Operator3/1 -> advPop/1
  Logical Operator4/1 -> pop/1
  Logical Operator8/1 -> Delay/1
  Relational Operator/1 -> Logical Operator2/2
  Relational Operator1/1 -> Delay8/1
  Relational Operator2/1 -> Logical Operator1/2
  Relational Operator3/1 -> Delay1/1
  Unit Delay Enabled Synchronous/1 -> Logical Operator4/2
  Unit Delay Enabled Synchronous1/1 -> Logical Operator3/2

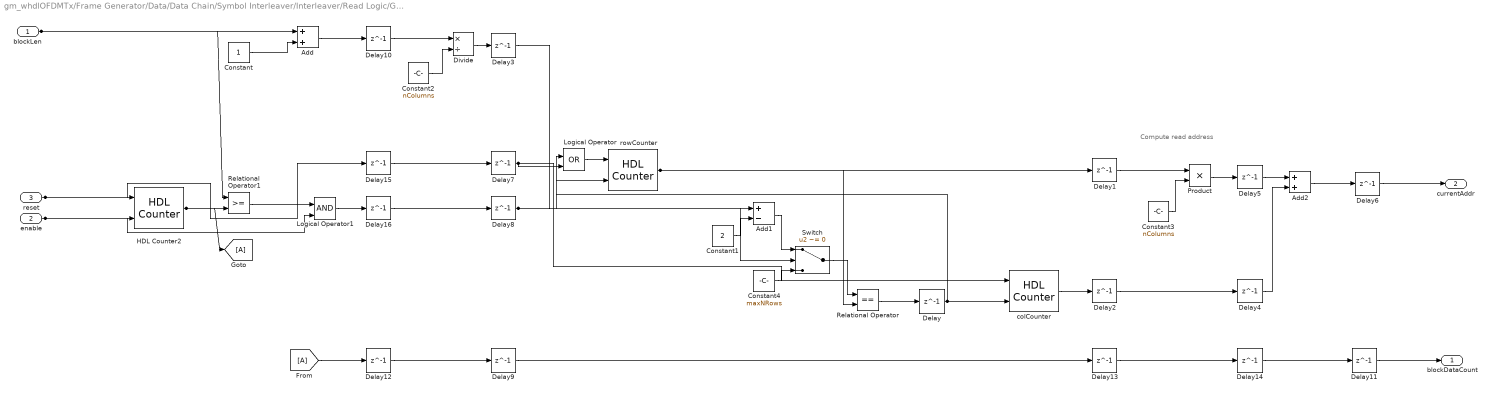
== system gm_whdlOFDMTx/Frame Generator/Data/Data Chain/Symbol Interleaver/Interleaver/Read Logic/Generate Read Address ==
  note: Compute read address
  blockLen : Inport  OutDataTypeStr=fixdt(0, 9, 0)  PortDimensions=1  SampleTime=2.44140625e-07
  enable : Inport  Port=2  OutDataTypeStr=boolean  PortDimensions=1  SampleTime=2.44140625e-07
  reset : Inport  Port=3  OutDataTypeStr=boolean  PortDimensions=1  SampleTime=2.44140625e-07
  Add : Sum
  Add1 : Sum  Inputs=+-  OutDataTypeStr=Inherit: Inherit via back propagation
  Add2 : Sum  OutDataTypeStr=fixdt(0,nextpow2(maxBlkSize),0)
  Constant : Constant  OutDataTypeStr=fixdt(0,1,0)  SampleTime=-1
  Constant1 : Constant  Value=2  OutDataTypeStr=fixdt(0,2,0)  SampleTime=-1
  Constant2 : Constant  Value=nColumns  OutDataTypeStr=fixdt(0,nextpow2(nColumns+1),0)  SampleTime=-1
  Constant3 : Constant  Value=nColumns  OutDataTypeStr=fixdt(0,nextpow2(nColumns+1),0)  SampleTime=-1
  Constant4 : Constant  Value=maxNRows  OutDataTypeStr=Inherit: Inherit via back propagation  SampleTime=-1
  Delay{,1..16} (17 alike) : Delay  DelayLength=1
  Divide : Product  Inputs=*/  OutDataTypeStr=fixdt(0,nextpow2(maxNRows+1),0)  RndMeth=Zero  SaturateOnIntegerOverflow=on
  From : From
  Goto : Goto
  HDL Counter2 : hdlsllib/Sources/HDL Counter  CountType=Count limited  CountInit=0  CountStep=1  CountMax=maxBlkSize  CountFromType=Initial value  CountFrom=0  CountResetPort=on  CountLoadPort=off  CountEnbPort=on  CountDirPort=off  CountHitOutputPort=off  CountDataType=Unsigned  CountWordLen=nextpow2(maxBlkSize+1)  CountFracLen=0  CountSampTime=1
  Logical Operator : Logic  Operator=OR  IconShape=distinctive  AllPortsSameDT=off  OutDataTypeStr=boolean
  Logical Operator1 : Logic  IconShape=distinctive  AllPortsSameDT=off  OutDataTypeStr=boolean
  Product : Product  OutDataTypeStr=fixdt(0,nextpow2(maxBlkSize),0)
  Relational Operator : RelationalOperator  Operator===  OutDataTypeStr=boolean  InputSameDT=off
  Relational Operator1 : RelationalOperator  OutDataTypeStr=boolean  InputSameDT=off
  Switch : Switch  Criteria=u2 ~= 0  SaturateOnIntegerOverflow=off  InputSameDT=off
  colCounter : hdlsllib/Sources/HDL Counter  CountType=Count limited  CountInit=0  CountStep=1  CountMax=nColumns -1  CountFromType=Initial value  CountFrom=0  CountResetPort=on  CountLoadPort=off  CountEnbPort=on  CountDirPort=off  CountHitOutputPort=off  CountDataType=Unsigned  CountWordLen=nextpow2(nColumns)  CountFracLen=0  CountSampTime=1
  rowCounter : hdlsllib/Sources/HDL Counter  CountType=Count limited  CountInit=0  CountStep=1  CountMax=maxNRows -1  CountFromType=Initial value  CountFrom=0  CountResetPort=on  CountLoadPort=off  CountEnbPort=on  CountDirPort=off  CountHitOutputPort=off  CountDataType=Unsigned  CountWordLen=nextpow2(maxNRows+1)  CountFracLen=0  CountSampTime=1
  blockDataCount : Outport  SampleTime=2.44140625e-07
  currentAddr : Outport  Port=2  SampleTime=2.44140625e-07
  wires:
  blockLen/1 -> Relational Operator1/1, Add/1
  enable/1 -> Logical Operator1/2, HDL Counter2/2
  reset/1 -> Delay15/1, HDL Counter2/1
  Add/1 -> Delay10/1
  Add1/1 -> Switch/1
  Add2/1 -> Delay6/1
  Constant/1 -> Add/2
  Constant1/1 -> Add1/2
  Constant2/1 -> Divide/2
  Constant3/1 -> Product/2
  Constant4/1 -> Switch/3
  Delay/1 -> Logical Operator/1, colCounter/2
  Delay1/1 -> Product/1
  Delay10/1 -> Divide/1
  Delay11/1 -> blockDataCount/1
  Delay12/1 -> Delay9/1
  Delay13/1 -> Delay14/1
  Delay14/1 -> Delay11/1
  Delay15/1 -> Delay7/1
  Delay16/1 -> Delay8/1
  Delay2/1 -> Delay4/1
  Delay3/1 -> Add1/1
  Delay4/1 -> Add2/2
  Delay5/1 -> Add2/1
  Delay6/1 -> currentAddr/1
  Delay7/1 -> Logical Operator/2, colCounter/1
  Delay8/1 -> Switch/2, rowCounter/2
  Delay9/1 -> Delay13/1
  Divide/1 -> Delay3/1
  From/1 -> Delay12/1
  HDL Counter2/1 -> Relational Operator1/2, Goto/1
  Logical Operator/1 -> rowCounter/1
  Logical Operator1/1 -> Delay16/1
  Product/1 -> Delay5/1
  Relational Operator/1 -> Delay/1
  Relational Operator1/1 -> Logical Operator1/1
  Switch/1 -> Relational Operator/1
  colCounter/1 -> Delay2/1
  rowCounter/1 -> Relational Operator/2, Delay1/1

== system gm_whdlOFDMTx/Frame Generator/Data/Data Chain/Symbol Interleaver/Interleaver/Read Logic/MATLAB Function ==
  trigger : Inport  OutDataTypeStr=boolean  PortDimensions=1  SampleTime=2.44140625e-07
  MATLAB Function : MATLAB Function  TreatAsAtomicUnit=on  mask{nClocks=maxBlkSize}
      mask prompts: nClocks "Number of clocks to hold:"
  out : Outport  SampleTime=2.44140625e-07  VectorParamsAs1DForOutWhenUnconnected=off
  wires:
  trigger/1 -> MATLAB Function/1(trigger)
  MATLAB Function/1(out) -> out/1

== system gm_whdlOFDMTx/Frame Generator/Data/Data Chain/Symbol Interleaver/Interleaver/Write Logic/Generate Write Address ==
  rst : Inport  OutDataTypeStr=boolean  PortDimensions=1  SampleTime=2.44140625e-07
  enb : Inport  Port=2  OutDataTypeStr=boolean  PortDimensions=1  SampleTime=2.44140625e-07
  end : Inport  Port=3  OutDataTypeStr=boolean  PortDimensions=1  SampleTime=2.44140625e-07
  Add : Sum  OutDataTypeStr=Inherit: Inherit via back propagation
  Constant : Constant  Value=0  OutDataTypeStr=fixdt(0,nextpow2(maxBlkSize+1),0)  SampleTime=-1
  Constant4 : Constant  Value=maxBlkSize  OutDataTypeStr=fixdt(0,nextpow2(maxBlkSize+1),0)  SampleTime=-1
  HDL Counter : hdlsllib/Sources/HDL Counter  CountType=Count limited  CountInit=0  CountStep=1  CountMax=maxBlkSize  CountFromType=Initial value  CountFrom=0  CountResetPort=on  CountLoadPort=off  CountEnbPort=on  CountDirPort=off  CountHitOutputPort=off  CountDataType=Unsigned  CountWordLen=nextpow2(maxBlkSize+1)  CountFracLen=0  CountSampTime=1
  Logical Operator7 : Logic  Operator=NOT  IconShape=distinctive  AllPortsSameDT=off  OutDataTypeStr=boolean
  Switch : Switch  Criteria=u2 ~= 0  SaturateOnIntegerOverflow=off  InputSameDT=off
  Unit Delay Enabled Synchronous2 : hdlsllib/Discrete/Unit Delay Enabled Synchronous  InitialCondition=0  SampleTime=-1
  wrAddr : Outport  SampleTime=2.44140625e-07
  count : Outport  Port=2  SampleTime=2.44140625e-07
  wires:
  rst/1 -> HDL Counter/1
  enb/1 -> HDL Counter/2
  end/1 -> Unit Delay Enabled Synchronous2/2
  Add/1 -> wrAddr/1
  Constant/1 -> Switch/3
  Constant4/1 -> Switch/1
  HDL Counter/1 -> Add/1, count/1
  Logical Operator7/1 -> Unit Delay Enabled Synchronous2/1
  Switch/1 -> Add/2
  Unit Delay Enabled Synchronous2/1 -> Switch/2, Logical Operator7/1

== system gm_whdlOFDMTx/Frame Generator/Data/Data Chain/Symbol Interleaver/Interleaver/Write Logic/Handle Input Control Signals ==
  start : Inport  OutDataTypeStr=boolean  PortDimensions=1  SampleTime=2.44140625e-07
  valid : Inport  Port=2  OutDataTypeStr=boolean  PortDimensions=1  SampleTime=2.44140625e-07
  end : Inport  Port=3  OutDataTypeStr=boolean  PortDimensions=1  SampleTime=2.44140625e-07
  Delay{1..5} (5 alike) : Delay  DelayLength=1
  Generate Current Frame Status : Subsystem
  Generate Forced End : Subsystem
  Logical Operator : Logic  Operator=OR  IconShape=distinctive  AllPortsSameDT=off  OutDataTypeStr=boolean
  Logical Operator1 : Logic  Operator=NOT  IconShape=distinctive  AllPortsSameDT=off  OutDataTypeStr=boolean
  Logical Operator2 : Logic  IconShape=distinctive  AllPortsSameDT=off  OutDataTypeStr=boolean
  Logical Operator3 : Logic  Inputs=4  IconShape=distinctive  AllPortsSameDT=off  OutDataTypeStr=boolean
  Logical Operator5 : Logic  IconShape=distinctive  AllPortsSameDT=off  OutDataTypeStr=boolean
  reset : Outport  SampleTime=2.44140625e-07
  countEnb : Outport  Port=2  SampleTime=2.44140625e-07
  endOut : Outport  Port=3  SampleTime=2.44140625e-07
  endReady : Outport  Port=4  SampleTime=2.44140625e-07
  wires:
  start/1 -> Logical Operator2/1
  valid/1 -> Logical Operator3/1, Logical Operator2/2, Delay4/1, Generate Forced End/2(valid)
  end/1 -> Logical Operator3/2
  Delay1/1 -> Logical Operator1/1, Delay5/1, Generate Current Frame Status/2(end)
  Delay2/1 -> reset/1
  Delay3/1 -> countEnb/1
  Delay4/1 -> Logical Operator5/1
  Delay5/1 -> endOut/1
  Generate Current Frame Status/1(frameOn) -> Logical Operator5/2, Logical Operator3/3, Generate Forced End/3(frameOn)
  Generate Forced End/1(forcedEnd) -> Logical Operator/2
  Logical Operator/1 -> Delay1/1, endReady/1
  Logical Operator1/1 -> Logical Operator3/4
  Logical Operator2/1 -> Delay2/1, Generate Current Frame Status/1(start), Generate Forced End/1(rst)
  Logical Operator3/1 -> Logical Operator/1
  Logical Operator5/1 -> Delay3/1

== system gm_whdlOFDMTx/Frame Generator/Data/Data Chain/Symbol Interleaver/Interleaver/Write Logic/Handle Input Control Signals/Generate Current Frame Status ==
  start : Inport  OutDataTypeStr=boolean  PortDimensions=1  SampleTime=2.44140625e-07
  end : Inport  Port=2  OutDataTypeStr=boolean  PortDimensions=1  SampleTime=2.44140625e-07
  Constant2 : Constant  Value=true  OutDataTypeStr=Inherit: Inherit via back propagation  SampleTime=-1
  Constant3 : Constant  Value=false  OutDataTypeStr=Inherit: Inherit via back propagation  SampleTime=-1
  Delay3 : Delay  DelayLength=1
  Logical Operator4 : Logic  Operator=OR  IconShape=distinctive  AllPortsSameDT=off  OutDataTypeStr=boolean
  Logical Operator6 : Logic  IconShape=distinctive  AllPortsSameDT=off  OutDataTypeStr=boolean
  Logical Operator7 : Logic  Operator=NOT  IconShape=distinctive  AllPortsSameDT=off  OutDataTypeStr=boolean
  Switch2 : Switch  Criteria=u2 ~= 0  SaturateOnIntegerOverflow=off  InputSameDT=off
  Unit Delay Enabled Synchronous1 : hdlsllib/Discrete/Unit Delay Enabled Synchronous  InitialCondition=0  SampleTime=-1
  frameOn : Outport  SampleTime=2.44140625e-07
  wires:
  start/1 -> Switch2/2, Logical Operator4/1, Delay3/1
  end/1 -> Logical Operator6/2
  Constant2/1 -> Switch2/1
  Constant3/1 -> Switch2/3
  Delay3/1 -> Logical Operator7/1
  Logical Operator4/1 -> Unit Delay Enabled Synchronous1/2
  Logical Operator6/1 -> Logical Operator4/2
  Logical Operator7/1 -> Logical Operator6/1
  Switch2/1 -> Unit Delay Enabled Synchronous1/1
  Unit Delay Enabled Synchronous1/1 -> frameOn/1

== system gm_whdlOFDMTx/Frame Generator/Data/Data Chain/Symbol Interleaver/Interleaver/Write Logic/Handle Input Control Signals/Generate Forced End ==
  rst : Inport  OutDataTypeStr=boolean  PortDimensions=1  SampleTime=2.44140625e-07
  valid : Inport  Port=2  OutDataTypeStr=boolean  PortDimensions=1  SampleTime=2.44140625e-07
  frameOn : Inport  Port=3  OutDataTypeStr=boolean  PortDimensions=1  SampleTime=2.44140625e-07
  Compare To Constant1 : simulink/Logic and Bit Operations/Compare To Constant  relop===  const=maxBlkSize -2  OutDataTypeStr=boolean
  Logical Operator1 : Logic  IconShape=distinctive  AllPortsSameDT=off  OutDataTypeStr=boolean
  Logical Operator6 : Logic  IconShape=distinctive  AllPortsSameDT=off  OutDataTypeStr=boolean
  readyCounter : hdlsllib/Sources/HDL Counter  CountType=Count limited  CountInit=0  CountStep=1  CountMax=maxBlkSize  CountFromType=Initial value  CountFrom=0  CountResetPort=on  CountLoadPort=off  CountEnbPort=on  CountDirPort=off  CountHitOutputPort=off  CountDataType=Unsigned  CountWordLen=nextpow2(maxBlkSize+1)  CountFracLen=0  CountSampTime=1
  forcedEnd : Outport  SampleTime=2.44140625e-07
  wires:
  rst/1 -> readyCounter/1
  valid/1 -> Logical Operator1/1
  frameOn/1 -> Logical Operator1/2
  Compare To Constant1/1 -> Logical Operator6/1
  Logical Operator1/1 -> Logical Operator6/2, readyCounter/2
  Logical Operator6/1 -> forcedEnd/1
  readyCounter/1 -> Compare To Constant1/1

== matlab function gm_whdlOFDMTx/Frame Generator/Data/Data and Control Signal Generation/Select Puncture Vector/Select Puncture Vector ==
  data: codeRate input; puncVec output
function puncVec = selPuncVec(codeRate)
%#codegen

persistent vector

if(isempty(vector))
vector = logical([1 1 1 1 1 1 1 1 1 1;
                  0 0 0 0 0 0 1 1 0 1;
                  0 0 0 0 1 1 1 0 0 1;
                  1 1 1 0 0 1 1 0 0 1]');
end
       
puncVec = vector(:,fi(codeRate+1,0,3,0));

end

== matlab function gm_whdlOFDMTx/Frame Formation and OFDM Modulation/Generate OFDM Modulator Valid/Counter for Read Address/Counter for Read Address ==
  data: out output fixdt(0,wordLength,0); enableIn input; wordLength parameter; initValue parameter; finalValue parameter
function out = counter(enableIn,wordLength, initValue, finalValue)
%#codegen

persistent tempOut

if(isempty(tempOut))
    tempOut = fi(initValue,0,wordLength,0);
end

if(enableIn)
    if(tempOut(:) == finalValue)
        tempOut(:) = initValue;
    else
        tempOut(:) = tempOut+1;
    end
end

out = tempOut;

end

== matlab function gm_whdlOFDMTx/Frame Generator/Data/Data Chain/Symbol Interleaver/Interleaver/Generate Ready/MATLAB Function1/MATLAB Function1 ==
  data: trigger input; out output; nClocks parameter
function out = holdPulse(trigger,nClocks)
%#codegen

 persistent count state;
 if isempty(count)
     count = fi(0,0,nextpow2(nClocks+2),0,hdlfimath);
     state = false;
 end
 
 
 %% Executes in current clock cycle
 if trigger
     state = true;
     count(:) = 0;
 end
 
 if(state && ~trigger)
     count(:) = count +1;
 end
 
 if(count(:) == (nClocks))
    state = false;
 end
     
 out = state;
 
end

== matlab function gm_whdlOFDMTx/Frame Generator/Data/Data Chain/Symbol Interleaver/Interleaver/Read Logic/MATLAB Function/MATLAB Function ==
  data: trigger input; out output; nClocks parameter
function out = holdPulse(trigger,nClocks)
%#codegen

 persistent count state;
 if isempty(count)
     count = fi(0,0,nextpow2(nClocks+1),0,hdlfimath);
     state = false;
 end
 
 %% Executes in next clock cycle
 if(count(:) == (nClocks))
    state = false;
 end
     
 out = state;
 
 
 %% Executes in current clock cycle
 if trigger
     state = true;
     count(:) = 0;
 end
 
 if(state && ~trigger)
     count(:) = count +1;
 end
 
end

== matlab function gm_whdlOFDMTx/Frame Generator/Header/Interleaver/Generate Ready/MATLAB Function1/MATLAB Function1 ==
  data: trigger input; out output; nClocks parameter
function out = holdPulse(trigger,nClocks)
%#codegen

 persistent count state;
 if isempty(count)
     count = fi(0,0,nextpow2(nClocks+2),0,hdlfimath);
     state = false;
 end
 
 
 %% Executes in current clock cycle
 if trigger
     state = true;
     count(:) = 0;
 end
 
 if(state && ~trigger)
     count(:) = count +1;
 end
 
 if(count(:) == (nClocks))
    state = false;
 end
     
 out = state;
 
end

== matlab function gm_whdlOFDMTx/Frame Generator/Header/Interleaver/Read Logic/MATLAB Function/MATLAB Function ==
  data: trigger input; out output; nClocks parameter
function out = holdPulse(trigger,nClocks)
%#codegen

 persistent count state;
 if isempty(count)
     count = fi(0,0,nextpow2(nClocks+1),0,hdlfimath);
     state = false;
 end
 
 %% Executes in next clock cycle
 if(count(:) == (nClocks))
    state = false;
 end
     
 out = state;
 
 
 %% Executes in current clock cycle
 if trigger
     state = true;
     count(:) = 0;
 end
 
 if(state && ~trigger)
     count(:) = count +1;
 end
 
end

== matlab function gm_whdlOFDMTx/Frame Controller and Input Sampler/Frame Controller/Generate OFDM Modulator Ready/MATLAB Function1/MATLAB Function1 ==
  data: trigger input; out output; nClocks parameter
function out = holdPulse(trigger,nClocks)
%#codegen

 persistent count state;
 if isempty(count)
     count = fi(0,0,nextpow2(nClocks+1),0,hdlfimath);
     state = false;
 end
 
 %% Executes in next clock cycle
 if(count(:) == (nClocks))
    state = false;
 end
     
 out = state;
 
 
 %% Executes in current clock cycle
 if trigger
     state = true;
     count(:) = 0;
 end
 
 if(state && ~trigger)
     count(:) = count +1;
 end
 
end

== matlab function gm_whdlOFDMTx/Frame Controller and Input Sampler/Frame Controller/Generate OFDM Modulator Ready/Control OFDM Signal Generation/MATLAB Function2/MATLAB Function2 ==
  data: trigger input; out output; nClocks parameter
function out = holdPulse(trigger,nClocks)
%#codegen

 persistent count state;
 if isempty(count)
     count = fi(0,0,nextpow2(nClocks+1),0,hdlfimath);
     state = false;
 end
 
 %% Executes in next clock cycle
 if(count(:) == (nClocks))
    state = false;
 end
     
 out = state;
 
 
 %% Executes in current clock cycle
 if trigger
     state = true;
     count(:) = 0;
 end
 
 if(state && ~trigger)
     count(:) = count +1;
 end
 
end

== matlab function gm_whdlOFDMTx/Frame Controller and Input Sampler/Enable Header and Preamble /MATLAB Function3/MATLAB Function3 ==
  data: trigger input; out output; nClocks parameter
function out = holdPulse(trigger,nClocks)
%#codegen

 persistent count state;
 if isempty(count)
     count = fi(0,0,nextpow2(nClocks+1),0,hdlfimath);
     state = false;
 end
 
 %% Executes in next clock cycle
 if(count(:) == (nClocks))
    state = false;
 end
     
 out = state;
 
 
 %% Executes in current clock cycle
 if trigger
     state = true;
     count(:) = 0;
 end
 
 if(state && ~trigger)
     count(:) = count +1;
 end
 
end

== matlab function gm_whdlOFDMTx/Frame Controller and Input Sampler/Enable Header and Preamble /MATLAB Function4/MATLAB Function4 ==
  data: trigger input; out output; nClocks parameter
function out = holdPulse(trigger,nClocks)
%#codegen

 persistent count state;
 if isempty(count)
     count = fi(0,0,nextpow2(nClocks+1),0,hdlfimath);
     state = false;
 end
 
 %% Executes in next clock cycle
 if(count(:) == (nClocks))
    state = false;
 end
     
 out = state;
 
 
 %% Executes in current clock cycle
 if trigger
     state = true;
     count(:) = 0;
 end
 
 if(state && ~trigger)
     count(:) = count +1;
 end
 
end

== matlab function gm_whdlOFDMTx/Multiplexer/Multiplex Preamble Signals/Priority Encoder/Priority Encoder ==
  data: ssValid input; selLine output; rsValid input; pilotValid input
function selLine = selectSignal(ssValid,rsValid,pilotValid)
%#codegen
if(ssValid)
    selLine = fi(0,0,3,0);
elseif(rsValid)
    selLine = fi(1,0,3,0);
elseif(pilotValid)
    selLine = fi(2,0,3,0);
else
    selLine = fi(0,0,3,0);
end

end

== matlab function gm_whdlOFDMTx/Frame Controller and Input Sampler/Frame Controller/Generate OFDM Modulator Ready/Control OFDM Signal Generation/Disable OFDM Generation/MATLAB Function5/MATLAB Function5 ==
  data: trigger input; out output; nClocks parameter
function out = holdPulseZeroLatency(trigger,nClocks)
%#codegen

 persistent count state;
 if isempty(count)
     count = fi(0,0,nextpow2(nClocks+1),0,hdlfimath);
     state = false;
 end
 
 %% Executes in single clock cycle
 if trigger
     state = true;
     count(:) = 0;
 end
 
 if(state && ~trigger)
     count(:) = count +1;
 end
 
 if(count(:) == (nClocks))
    state = false;
 end
     
 out = state;
 
end
